simulink model "walkingRobotRL3D"  (R2020b)
settings: Solver=ode23t  StartTime=0.0  StopTime=Tf  RelTol=1e-2  EnableMultiTasking=on
PreLoadFcn:
  | robotParametersRL
undefined symbols (not defined in the file): agent, ankleD_pitch_jointMAX, ankleD_pitch_jointMIN, ankleD_roll_jointMAX, ankleD_roll_jointMIN, ankleI_pitch_jointMAX, ankleI_pitch_jointMIN, ankleI_roll_jointMAX, ankleI_roll_jointMIN, getSampleTime, height_plane, hipD_pitch_jointMAX, hipD_pitch_jointMIN, hipD_roll_jointMAX, hipD_roll_jointMIN, hipI_pitch_jointMAX, hipI_pitch_jointMIN, hipI_roll_jointMAX, hipI_roll_jointMIN, init_angs_L, init_angs_R, init_height, joint_damping, joint_limit_damping, joint_limit_stiffness, joint_stiffness, kneeD_jointMAX, kneeD_jointMIN, kneeI_jointMAX, kneeI_jointMIN, lower_leg_I0, lower_leg_length, lower_leg_mass, lower_leg_x, lower_leg_y, muscle_nominal_length, p10_ankleD_roll, plane_x, plane_y, regulator_type, tau, Tf, torso_height, torso_length, torso_offset_x, torso_offset_z, torso_width, torso_x, torso_y, torso_z, Ts, upper_leg_I0, upper_leg_length, upper_leg_mass, upper_leg_x, upper_leg_y, v10_ankleD_pitch, v10_ankleD_roll, v10_ankleI_pitch, v10_ankleI_roll ... (+41)
libraries: sm_lib x222, simulink x183, nesl_utility x130, walkingRobotUtils x69, rllib x2
(part 13 of 24)

== system walkingRobotRL3D/Walking Robot2/Robot Leg R1/Knee Joint ==
  t : Inport
  Bus Creator : BusCreator  Inputs=3
  PS-Simulink Converter1 : nesl_utility/PS-Simulink Converter  PhysicalDomain=network_engine_domain  SubClassName=ps_output  LeftPortType=input  RightPortType=output  PseudoPeriodic=off  Frequencies=[]  Unit=N*m  AffineConversion=off
  PS-Simulink Converter2 : nesl_utility/PS-Simulink Converter  PhysicalDomain=network_engine_domain  SubClassName=ps_output  LeftPortType=input  RightPortType=output  PseudoPeriodic=off  Frequencies=[]  Unit=rad/s  AffineConversion=off
  Revolute Joint : sm_lib/Joints/Revolute Joint  JointMode=Normal  SenseConstraintForce=off  SenseConstraintForceX=off  SenseConstraintForceY=off  SenseConstraintForceZ=off  SenseConstraintTorque=off  SenseConstraintTorqueX=off  SenseConstraintTorqueY=off  SenseConstraintTorqueZ=off  SenseTotalForce=off  SenseTotalForceX=off  SenseTotalForceY=off  SenseTotalForceZ=off  SenseTotalTorque=off  SenseTotalTorqueX=off  SenseTotalTorqueY=off  SenseTotalTorqueZ=off  CompositeWrenchDir=FollowerOnBase  CompositeWrenchFrame=BaseFrame  EquilibriumPosition=eqAngle  EquilibriumPositionUnits=rad  SpringStiffness=k  SpringStiffnessUnits=N*m/rad  DampingCoefficient=d  DampingCoefficientUnits=N*m/(rad/s)  TorqueActuationMode=ComputedTorque  MotionActuationMode=InputMotion  SensePosition=off  SenseVelocity=on  SenseAcceleration=off  SenseTorqueForce=on  SenseLowerLimitTorqueForce=off  SenseUpperLimitTorqueForce=off  LowerLimitSpecify=on  LowerLimitBound=lowerLimit  LowerLimitBoundUnits=rad  LowerLimitStiffness=jointLimitStiffness  LowerLimitStiffnessUnits=N*m/rad  LowerLimitDamping=jointLimitDamping  LowerLimitDampingUnits=N*m/(rad/s)  LowerLimitTransitionRegionWidth=1  LowerLimitTransitionRegionWidthUnits=deg  UpperLimitSpecify=on  UpperLimitBound=upperLimit  UpperLimitBoundUnits=rad  UpperLimitStiffness=jointLimitStiffness  UpperLimitStiffnessUnits=N*m/rad  UpperLimitDamping=jointLimitDamping  UpperLimitDampingUnits=N*m/(rad/s)  UpperLimitTransitionRegionWidth=1  UpperLimitTransitionRegionWidthUnits=deg  PositionTargetSpecify=on  PositionTargetPriority=High  PositionTargetValue=initAngle  PositionTargetValueUnits=rad  VelocityTargetSpecify=off  VelocityTargetPriority=High  VelocityTargetValue=0  VelocityTargetValueUnits=deg/s
  Simulink-PS Converter : nesl_utility/Simulink-PS Converter  PhysicalDomain=network_engine_domain  SubClassName=ps_input  LeftPortType=input  RightPortType=output  PseudoPeriodic=off  Frequencies=[]  NoiseDistribution=none  NoiseParameters=[]  Unit=rad  AffineConversion=off  FilteringAndDerivatives=filter  SimscapeFilterOrder=2  InputFilterTimeConstant=motion_time_constant  UdotUserProvided=0
  B : PMIOPort  Side=Left
  F : PMIOPort  Port=2  Side=Right
  meas : Outport  VectorParamsAs1DForOutWhenUnconnected=off
  wires:
  PS-Simulink Converter1/1 -> Bus Creator/2  "torque"
  Bus Creator/1 -> meas/1
  t/1 -> Bus Creator/1, Simulink-PS Converter/1  "angle"
  PS-Simulink Converter2/1 -> Bus Creator/3  "speed"
  connections:
  Revolute Joint/LConn1 -- B/RConn1
  Revolute Joint/RConn1 -- F/RConn1
  Simulink-PS Converter/RConn1 -- Revolute Joint/LConn2
  Revolute Joint/RConn2 -- PS-Simulink Converter2/LConn1
  Revolute Joint/RConn3 -- PS-Simulink Converter1/LConn1

== system walkingRobotRL3D/Walking Robot2/Sensors/Calculate Actuator Power 3D ==
  meas : Inport
  Add : Sum  Inputs=5
  Bus Selector : BusSelector  OutputSignals=ankle_roll_angle,ankle_roll_speed,ankle_pitch_angle,ankle_pitch_speed,knee_angle,knee_speed,hip_roll_angle,hip_roll_speed,hip_pitch_angle,hip_pitch_speed
  Product{,1..4} (5 alike) : Product
  P : Outport  VectorParamsAs1DForOutWhenUnconnected=off
  wires:
  meas/1 -> Bus Selector/1
  Product2/1 -> Add/4
  Product1/1 -> Add/2
  Product/1 -> Add/1
  Add/1 -> P/1
  Bus Selector/1 -> Product/1  "<ankle_roll_angle>"
  Bus Selector/2 -> Product/2  "<ankle_roll_speed>"
  Bus Selector/3 -> Product1/1  "<ankle_pitch_angle>"
  Bus Selector/4 -> Product1/2  "<ankle_pitch_speed>"
  Bus Selector/5 -> Product3/1  "<knee_angle>"
  Bus Selector/6 -> Product3/2  "<knee_speed>"
  Bus Selector/7 -> Product2/1  "<hip_roll_angle>"
  Bus Selector/8 -> Product2/2  "<hip_roll_speed>"
  Bus Selector/10 -> Product4/2  "<hip_pitch_speed>"
  Bus Selector/9 -> Product4/1  "<hip_pitch_angle>"
  Product4/1 -> Add/5
  Product3/1 -> Add/3

== system walkingRobotRL3D/Walking Robot2/Sensors/Calculate Actuator Power 3D1 ==
  meas : Inport
  Add : Sum  Inputs=5
  Bus Selector : BusSelector  OutputSignals=ankle_roll_angle,ankle_roll_speed,ankle_pitch_angle,ankle_pitch_speed,knee_angle,knee_speed,hip_roll_angle,hip_roll_speed,hip_pitch_angle,hip_pitch_speed
  Product{,1..4} (5 alike) : Product
  P : Outport  VectorParamsAs1DForOutWhenUnconnected=off
  wires:
  Product3/1 -> Add/3
  Product4/1 -> Add/5
  Bus Selector/9 -> Product4/1  "<hip_pitch_angle>"
  Bus Selector/10 -> Product4/2  "<hip_pitch_speed>"
  Bus Selector/8 -> Product2/2  "<hip_roll_speed>"
  Bus Selector/7 -> Product2/1  "<hip_roll_angle>"
  Bus Selector/6 -> Product3/2  "<knee_speed>"
  Bus Selector/5 -> Product3/1  "<knee_angle>"
  Bus Selector/4 -> Product1/2  "<ankle_pitch_speed>"
  Bus Selector/3 -> Product1/1  "<ankle_pitch_angle>"
  Bus Selector/2 -> Product/2  "<ankle_roll_speed>"
  Bus Selector/1 -> Product/1  "<ankle_roll_angle>"
  Add/1 -> P/1
  Product/1 -> Add/1
  Product1/1 -> Add/2
  Product2/1 -> Add/4
  meas/1 -> Bus Selector/1

== system walkingRobotRL3D/Walking Robot33/DYNAMIC MODEL OF PAM FOR LEFT LEG/Dynamic Model Antagonisitic PAM1 ==
  V1 : Inport
  V2 : Inport  Port=2
  Abs : Abs  Commented=through
  Constant : Constant
  Constant1 : Constant
  F(x,P) mode (Muscles 1) : MATLAB Function  TreatAsAtomicUnit=on
  F(x,P) mode (Muscles 1)1 : MATLAB Function  TreatAsAtomicUnit=on
  Proportional Regulator (Muscles 1) : MATLAB Function  TreatAsAtomicUnit=on
  Proportional Regulator (Muscles 2) : MATLAB Function  TreatAsAtomicUnit=on
  Spring and damping model : Subsystem
  F1 : Outport
  F2 : Outport  Port=2
  wires:
  Constant1/1 -> Proportional Regulator (Muscles 2)/2(reg_type)
  F(x,P) mode (Muscles 1)/1(F1) -> Spring and damping model/1(F1), F1/1
  Proportional Regulator (Muscles 2)/1(p1) -> Spring and damping model/4(P2), F(x,P) mode (Muscles 1)1/1(P2)
  Proportional Regulator (Muscles 1)/1(p1) -> Spring and damping model/3(P1), F(x,P) mode (Muscles 1)/1(P1)
  Spring and damping model/1(x2) -> F(x,P) mode (Muscles 1)1/2(x_muscle2)
  F(x,P) mode (Muscles 1)1/1(F2) -> Abs/1
  Constant/1 -> Proportional Regulator (Muscles 1)/2(reg_type)
  V2/1 -> Proportional Regulator (Muscles 2)/1(V1)
  V1/1 -> Proportional Regulator (Muscles 1)/1(V1)
  Abs/1 -> F2/1, Spring and damping model/2(F2)
  Spring and damping model/2(x1) -> F(x,P) mode (Muscles 1)/2(x_muscle1)

== system walkingRobotRL3D/Walking Robot33/DYNAMIC MODEL OF PAM FOR LEFT LEG/Dynamic Model Antagonisitic PAM2 ==
  V1 : Inport
  V2 : Inport  Port=2
  Abs : Abs  Commented=through
  Constant : Constant
  Constant1 : Constant
  F(x,P) mode (Muscles 1) : MATLAB Function  TreatAsAtomicUnit=on
  F(x,P) mode (Muscles 1)1 : MATLAB Function  TreatAsAtomicUnit=on
  Proportional Regulator (Muscles 1) : MATLAB Function  TreatAsAtomicUnit=on
  Proportional Regulator (Muscles 2) : MATLAB Function  TreatAsAtomicUnit=on
  Spring and damping model : Subsystem
  F1 : Outport
  F2 : Outport  Port=2
  wires:
  Constant1/1 -> Proportional Regulator (Muscles 2)/2(reg_type)
  F(x,P) mode (Muscles 1)/1(F1) -> Spring and damping model/1(F1), F1/1
  Proportional Regulator (Muscles 2)/1(p1) -> Spring and damping model/4(P2), F(x,P) mode (Muscles 1)1/1(P2)
  Proportional Regulator (Muscles 1)/1(p1) -> Spring and damping model/3(P1), F(x,P) mode (Muscles 1)/1(P1)
  Spring and damping model/1(x2) -> F(x,P) mode (Muscles 1)1/2(x_muscle2)
  F(x,P) mode (Muscles 1)1/1(F2) -> Abs/1
  Constant/1 -> Proportional Regulator (Muscles 1)/2(reg_type)
  V2/1 -> Proportional Regulator (Muscles 2)/1(V1)
  V1/1 -> Proportional Regulator (Muscles 1)/1(V1)
  Abs/1 -> F2/1, Spring and damping model/2(F2)
  Spring and damping model/2(x1) -> F(x,P) mode (Muscles 1)/2(x_muscle1)

== system walkingRobotRL3D/Walking Robot33/DYNAMIC MODEL OF PAM FOR LEFT LEG/Dynamic Model Antagonisitic PAM3 ==
  V1 : Inport
  V2 : Inport  Port=2
  Abs : Abs  Commented=through
  Constant : Constant
  Constant1 : Constant
  F(x,P) mode (Muscles 1) : MATLAB Function  TreatAsAtomicUnit=on
  F(x,P) mode (Muscles 1)1 : MATLAB Function  TreatAsAtomicUnit=on
  Proportional Regulator (Muscles 1) : MATLAB Function  TreatAsAtomicUnit=on
  Proportional Regulator (Muscles 2) : MATLAB Function  TreatAsAtomicUnit=on
  Spring and damping model : Subsystem
  F1 : Outport
  F2 : Outport  Port=2
  wires:
  Constant1/1 -> Proportional Regulator (Muscles 2)/2(reg_type)
  F(x,P) mode (Muscles 1)/1(F1) -> Spring and damping model/1(F1), F1/1
  Proportional Regulator (Muscles 2)/1(p1) -> Spring and damping model/4(P2), F(x,P) mode (Muscles 1)1/1(P2)
  Proportional Regulator (Muscles 1)/1(p1) -> Spring and damping model/3(P1), F(x,P) mode (Muscles 1)/1(P1)
  Spring and damping model/1(x2) -> F(x,P) mode (Muscles 1)1/2(x_muscle2)
  F(x,P) mode (Muscles 1)1/1(F2) -> Abs/1
  Constant/1 -> Proportional Regulator (Muscles 1)/2(reg_type)
  V2/1 -> Proportional Regulator (Muscles 2)/1(V1)
  V1/1 -> Proportional Regulator (Muscles 1)/1(V1)
  Abs/1 -> F2/1, Spring and damping model/2(F2)
  Spring and damping model/2(x1) -> F(x,P) mode (Muscles 1)/2(x_muscle1)

== system walkingRobotRL3D/Walking Robot33/DYNAMIC MODEL OF PAM FOR LEFT LEG/Dynamic Model Antagonisitic PAM4 ==
  V1 : Inport
  V2 : Inport  Port=2
  Abs : Abs  Commented=through
  Constant : Constant
  Constant1 : Constant
  F(x,P) mode (Muscles 1) : MATLAB Function  TreatAsAtomicUnit=on
  F(x,P) mode (Muscles 1)1 : MATLAB Function  TreatAsAtomicUnit=on
  Proportional Regulator (Muscles 1) : MATLAB Function  TreatAsAtomicUnit=on
  Proportional Regulator (Muscles 2) : MATLAB Function  TreatAsAtomicUnit=on
  Spring and damping model : Subsystem
  F1 : Outport
  F2 : Outport  Port=2
  wires:
  Constant1/1 -> Proportional Regulator (Muscles 2)/2(reg_type)
  F(x,P) mode (Muscles 1)/1(F1) -> Spring and damping model/1(F1), F1/1
  Proportional Regulator (Muscles 2)/1(p1) -> Spring and damping model/4(P2), F(x,P) mode (Muscles 1)1/1(P2)
  Proportional Regulator (Muscles 1)/1(p1) -> Spring and damping model/3(P1), F(x,P) mode (Muscles 1)/1(P1)
  Spring and damping model/1(x2) -> F(x,P) mode (Muscles 1)1/2(x_muscle2)
  F(x,P) mode (Muscles 1)1/1(F2) -> Abs/1
  Constant/1 -> Proportional Regulator (Muscles 1)/2(reg_type)
  V2/1 -> Proportional Regulator (Muscles 2)/1(V1)
  V1/1 -> Proportional Regulator (Muscles 1)/1(V1)
  Abs/1 -> F2/1, Spring and damping model/2(F2)
  Spring and damping model/2(x1) -> F(x,P) mode (Muscles 1)/2(x_muscle1)

== system walkingRobotRL3D/Walking Robot33/DYNAMIC MODEL OF PAM FOR LEFT LEG/Dynamic Model Antagonisitic PAM5 ==
  V1 : Inport
  V2 : Inport  Port=2
  Abs : Abs  Commented=through
  Constant : Constant
  Constant1 : Constant
  F(x,P) mode (Muscles 1) : MATLAB Function  TreatAsAtomicUnit=on
  F(x,P) mode (Muscles 1)1 : MATLAB Function  TreatAsAtomicUnit=on
  Proportional Regulator (Muscles 1) : MATLAB Function  TreatAsAtomicUnit=on
  Proportional Regulator (Muscles 2) : MATLAB Function  TreatAsAtomicUnit=on
  Spring and damping model : Subsystem
  F1 : Outport
  F2 : Outport  Port=2
  wires:
  Constant1/1 -> Proportional Regulator (Muscles 2)/2(reg_type)
  F(x,P) mode (Muscles 1)/1(F1) -> Spring and damping model/1(F1), F1/1
  Proportional Regulator (Muscles 2)/1(p1) -> Spring and damping model/4(P2), F(x,P) mode (Muscles 1)1/1(P2)
  Proportional Regulator (Muscles 1)/1(p1) -> Spring and damping model/3(P1), F(x,P) mode (Muscles 1)/1(P1)
  Spring and damping model/1(x2) -> F(x,P) mode (Muscles 1)1/2(x_muscle2)
  F(x,P) mode (Muscles 1)1/1(F2) -> Abs/1
  Constant/1 -> Proportional Regulator (Muscles 1)/2(reg_type)
  V2/1 -> Proportional Regulator (Muscles 2)/1(V1)
  V1/1 -> Proportional Regulator (Muscles 1)/1(V1)
  Abs/1 -> F2/1, Spring and damping model/2(F2)
  Spring and damping model/2(x1) -> F(x,P) mode (Muscles 1)/2(x_muscle1)

== system walkingRobotRL3D/Walking Robot33/DYNAMIC MODEL OF PAM FOR RIGHT LEG/Dynamic Model Antagonisitic PAM1 ==
  V1 : Inport
  V2 : Inport  Port=2
  Abs : Abs  Commented=through
  Constant : Constant
  Constant1 : Constant
  F(x,P) mode (Muscles 1) : MATLAB Function  TreatAsAtomicUnit=on
  F(x,P) mode (Muscles 1)1 : MATLAB Function  TreatAsAtomicUnit=on
  Proportional Regulator (Muscles 1) : MATLAB Function  TreatAsAtomicUnit=on
  Proportional Regulator (Muscles 2) : MATLAB Function  TreatAsAtomicUnit=on
  Spring and damping model : Subsystem
  F1 : Outport
  F2 : Outport  Port=2
  wires:
  Constant1/1 -> Proportional Regulator (Muscles 2)/2(reg_type)
  F(x,P) mode (Muscles 1)/1(F1) -> Spring and damping model/1(F1), F1/1
  Proportional Regulator (Muscles 2)/1(p1) -> Spring and damping model/4(P2), F(x,P) mode (Muscles 1)1/1(P2)
  Proportional Regulator (Muscles 1)/1(p1) -> Spring and damping model/3(P1), F(x,P) mode (Muscles 1)/1(P1)
  Spring and damping model/1(x2) -> F(x,P) mode (Muscles 1)1/2(x_muscle2)
  F(x,P) mode (Muscles 1)1/1(F2) -> Abs/1
  Constant/1 -> Proportional Regulator (Muscles 1)/2(reg_type)
  V2/1 -> Proportional Regulator (Muscles 2)/1(V1)
  V1/1 -> Proportional Regulator (Muscles 1)/1(V1)
  Abs/1 -> F2/1, Spring and damping model/2(F2)
  Spring and damping model/2(x1) -> F(x,P) mode (Muscles 1)/2(x_muscle1)

== system walkingRobotRL3D/Walking Robot33/DYNAMIC MODEL OF PAM FOR RIGHT LEG/Dynamic Model Antagonisitic PAM2 ==
  V1 : Inport
  V2 : Inport  Port=2
  Abs : Abs  Commented=through
  Constant : Constant
  Constant1 : Constant
  F(x,P) mode (Muscles 1) : MATLAB Function  TreatAsAtomicUnit=on
  F(x,P) mode (Muscles 1)1 : MATLAB Function  TreatAsAtomicUnit=on
  Proportional Regulator (Muscles 1) : MATLAB Function  TreatAsAtomicUnit=on
  Proportional Regulator (Muscles 2) : MATLAB Function  TreatAsAtomicUnit=on
  Spring and damping model : Subsystem
  F1 : Outport
  F2 : Outport  Port=2
  wires:
  Constant1/1 -> Proportional Regulator (Muscles 2)/2(reg_type)
  F(x,P) mode (Muscles 1)/1(F1) -> Spring and damping model/1(F1), F1/1
  Proportional Regulator (Muscles 2)/1(p1) -> Spring and damping model/4(P2), F(x,P) mode (Muscles 1)1/1(P2)
  Proportional Regulator (Muscles 1)/1(p1) -> Spring and damping model/3(P1), F(x,P) mode (Muscles 1)/1(P1)
  Spring and damping model/1(x2) -> F(x,P) mode (Muscles 1)1/2(x_muscle2)
  F(x,P) mode (Muscles 1)1/1(F2) -> Abs/1
  Constant/1 -> Proportional Regulator (Muscles 1)/2(reg_type)
  V2/1 -> Proportional Regulator (Muscles 2)/1(V1)
  V1/1 -> Proportional Regulator (Muscles 1)/1(V1)
  Abs/1 -> F2/1, Spring and damping model/2(F2)
  Spring and damping model/2(x1) -> F(x,P) mode (Muscles 1)/2(x_muscle1)

== system walkingRobotRL3D/Walking Robot33/DYNAMIC MODEL OF PAM FOR RIGHT LEG/Dynamic Model Antagonisitic PAM3 ==
  V1 : Inport
  V2 : Inport  Port=2
  Abs : Abs  Commented=through
  Constant : Constant
  Constant1 : Constant
  F(x,P) mode (Muscles 1) : MATLAB Function  TreatAsAtomicUnit=on
  F(x,P) mode (Muscles 1)1 : MATLAB Function  TreatAsAtomicUnit=on
  Proportional Regulator (Muscles 1) : MATLAB Function  TreatAsAtomicUnit=on
  Proportional Regulator (Muscles 2) : MATLAB Function  TreatAsAtomicUnit=on
  Spring and damping model : Subsystem
  F1 : Outport
  F2 : Outport  Port=2
  wires:
  Constant1/1 -> Proportional Regulator (Muscles 2)/2(reg_type)
  F(x,P) mode (Muscles 1)/1(F1) -> Spring and damping model/1(F1), F1/1
  Proportional Regulator (Muscles 2)/1(p1) -> Spring and damping model/4(P2), F(x,P) mode (Muscles 1)1/1(P2)
  Proportional Regulator (Muscles 1)/1(p1) -> Spring and damping model/3(P1), F(x,P) mode (Muscles 1)/1(P1)
  Spring and damping model/1(x2) -> F(x,P) mode (Muscles 1)1/2(x_muscle2)
  F(x,P) mode (Muscles 1)1/1(F2) -> Abs/1
  Constant/1 -> Proportional Regulator (Muscles 1)/2(reg_type)
  V2/1 -> Proportional Regulator (Muscles 2)/1(V1)
  V1/1 -> Proportional Regulator (Muscles 1)/1(V1)
  Abs/1 -> F2/1, Spring and damping model/2(F2)
  Spring and damping model/2(x1) -> F(x,P) mode (Muscles 1)/2(x_muscle1)

== system walkingRobotRL3D/Walking Robot33/DYNAMIC MODEL OF PAM FOR RIGHT LEG/Dynamic Model Antagonisitic PAM4 ==
  V1 : Inport
  V2 : Inport  Port=2
  Abs : Abs  Commented=through
  Constant : Constant
  Constant1 : Constant
  F(x,P) mode (Muscles 1) : MATLAB Function  TreatAsAtomicUnit=on
  F(x,P) mode (Muscles 1)1 : MATLAB Function  TreatAsAtomicUnit=on
  Proportional Regulator (Muscles 1) : MATLAB Function  TreatAsAtomicUnit=on
  Proportional Regulator (Muscles 2) : MATLAB Function  TreatAsAtomicUnit=on
  Spring and damping model : Subsystem
  F1 : Outport
  F2 : Outport  Port=2
  wires:
  Constant1/1 -> Proportional Regulator (Muscles 2)/2(reg_type)
  F(x,P) mode (Muscles 1)/1(F1) -> Spring and damping model/1(F1), F1/1
  Proportional Regulator (Muscles 2)/1(p1) -> Spring and damping model/4(P2), F(x,P) mode (Muscles 1)1/1(P2)
  Proportional Regulator (Muscles 1)/1(p1) -> Spring and damping model/3(P1), F(x,P) mode (Muscles 1)/1(P1)
  Spring and damping model/1(x2) -> F(x,P) mode (Muscles 1)1/2(x_muscle2)
  F(x,P) mode (Muscles 1)1/1(F2) -> Abs/1
  Constant/1 -> Proportional Regulator (Muscles 1)/2(reg_type)
  V2/1 -> Proportional Regulator (Muscles 2)/1(V1)
  V1/1 -> Proportional Regulator (Muscles 1)/1(V1)
  Abs/1 -> F2/1, Spring and damping model/2(F2)
  Spring and damping model/2(x1) -> F(x,P) mode (Muscles 1)/2(x_muscle1)

== system walkingRobotRL3D/Walking Robot33/DYNAMIC MODEL OF PAM FOR RIGHT LEG/Dynamic Model Antagonisitic PAM5 ==
  V1 : Inport
  V2 : Inport  Port=2
  Abs : Abs  Commented=through
  Constant : Constant
  Constant1 : Constant
  F(x,P) mode (Muscles 1) : MATLAB Function  TreatAsAtomicUnit=on
  F(x,P) mode (Muscles 1)1 : MATLAB Function  TreatAsAtomicUnit=on
  Proportional Regulator (Muscles 1) : MATLAB Function  TreatAsAtomicUnit=on
  Proportional Regulator (Muscles 2) : MATLAB Function  TreatAsAtomicUnit=on
  Spring and damping model : Subsystem
  F1 : Outport
  F2 : Outport  Port=2
  wires:
  Constant1/1 -> Proportional Regulator (Muscles 2)/2(reg_type)
  F(x,P) mode (Muscles 1)/1(F1) -> Spring and damping model/1(F1), F1/1
  Proportional Regulator (Muscles 2)/1(p1) -> Spring and damping model/4(P2), F(x,P) mode (Muscles 1)1/1(P2)
  Proportional Regulator (Muscles 1)/1(p1) -> Spring and damping model/3(P1), F(x,P) mode (Muscles 1)/1(P1)
  Spring and damping model/1(x2) -> F(x,P) mode (Muscles 1)1/2(x_muscle2)
  F(x,P) mode (Muscles 1)1/1(F2) -> Abs/1
  Constant/1 -> Proportional Regulator (Muscles 1)/2(reg_type)
  V2/1 -> Proportional Regulator (Muscles 2)/1(V1)
  V1/1 -> Proportional Regulator (Muscles 1)/1(V1)
  Abs/1 -> F2/1, Spring and damping model/2(F2)
  Spring and damping model/2(x1) -> F(x,P) mode (Muscles 1)/2(x_muscle1)

== system walkingRobotRL3D/Walking Robot33/Sensors/Calculate Actuator Power 3D ==
  meas : Inport
  Add : Sum  Inputs=5
  Bus Selector : BusSelector  OutputSignals=ankle_roll_angle,ankle_roll_speed,ankle_pitch_angle,ankle_pitch_speed,knee_angle,knee_speed,hip_roll_angle,hip_roll_speed,hip_pitch_angle,hip_pitch_speed
  Product{,1..4} (5 alike) : Product
  P : Outport  VectorParamsAs1DForOutWhenUnconnected=off
  wires:
  meas/1 -> Bus Selector/1
  Product2/1 -> Add/4
  Product1/1 -> Add/2
  Product/1 -> Add/1
  Add/1 -> P/1
  Bus Selector/1 -> Product/1  "<ankle_roll_angle>"
  Bus Selector/2 -> Product/2  "<ankle_roll_speed>"
  Bus Selector/3 -> Product1/1  "<ankle_pitch_angle>"
  Bus Selector/4 -> Product1/2  "<ankle_pitch_speed>"
  Bus Selector/5 -> Product3/1  "<knee_angle>"
  Bus Selector/6 -> Product3/2  "<knee_speed>"
  Bus Selector/7 -> Product2/1  "<hip_roll_angle>"
  Bus Selector/8 -> Product2/2  "<hip_roll_speed>"
  Bus Selector/10 -> Product4/2  "<hip_pitch_speed>"
  Bus Selector/9 -> Product4/1  "<hip_pitch_angle>"
  Product4/1 -> Add/5
  Product3/1 -> Add/3

== system walkingRobotRL3D/Walking Robot33/Sensors/Calculate Actuator Power 3D1 ==
  meas : Inport
  Add : Sum  Inputs=5
  Bus Selector : BusSelector  OutputSignals=ankle_roll_angle,ankle_roll_speed,ankle_pitch_angle,ankle_pitch_speed,knee_angle,knee_speed,hip_roll_angle,hip_roll_speed,hip_pitch_angle,hip_pitch_speed
  Product{,1..4} (5 alike) : Product
  P : Outport  VectorParamsAs1DForOutWhenUnconnected=off
  wires:
  Product3/1 -> Add/3
  Product4/1 -> Add/5
  Bus Selector/9 -> Product4/1  "<hip_pitch_angle>"
  Bus Selector/10 -> Product4/2  "<hip_pitch_speed>"
  Bus Selector/8 -> Product2/2  "<hip_roll_speed>"
  Bus Selector/7 -> Product2/1  "<hip_roll_angle>"
  Bus Selector/6 -> Product3/2  "<knee_speed>"
  Bus Selector/5 -> Product3/1  "<knee_angle>"
  Bus Selector/4 -> Product1/2  "<ankle_pitch_speed>"
  Bus Selector/3 -> Product1/1  "<ankle_pitch_angle>"
  Bus Selector/2 -> Product/2  "<ankle_roll_speed>"
  Bus Selector/1 -> Product/1  "<ankle_roll_angle>"
  Add/1 -> P/1
  Product/1 -> Add/1
  Product1/1 -> Add/2
  Product2/1 -> Add/4
  meas/1 -> Bus Selector/1

== system walkingRobotRL3D/Walking Robot/DYNAMIC MODEL OF PAM FOR LEFT LEG/Dynamic Model Antagonisitic PAM1/Spring and damping model ==
  F1 : Inport
  F2 : Inport  Port=2
  P1 : Inport  Port=3
  P2 : Inport  Port=4
  Dynamic muscle 2 : Subsystem
  Dynamics muscle 1 : Subsystem
  S(P),D(P) : MATLAB Function  TreatAsAtomicUnit=on
  Unit Delay : UnitDelay  SampleTime=-1  HasFrameUpgradeWarning=on
  Unit Delay1 : UnitDelay  SampleTime=-1  HasFrameUpgradeWarning=on
  Unit Delay2 : UnitDelay  Commented=through  SampleTime=-1  HasFrameUpgradeWarning=on
  Unit Delay3 : UnitDelay  Commented=through  SampleTime=-1  HasFrameUpgradeWarning=on
  x1(m)->x1(%) : Gain  Gain=100/muscle_nominal_length
  x2(m)->x2(%) : Gain  Gain=100/muscle_nominal_length
  x2 : Outport
  x1 : Outport  Port=2
  wires:
  Dynamics muscle 1/1(R1) -> Unit Delay/1
  F1/1 -> Unit Delay2/1
  Dynamic muscle 2/2(x2) -> x2(m)->x2(%)/1
  Dynamics muscle 1/2(x1) -> x1(m)->x1(%)/1
  P1/1 -> S(P),D(P)/1(P1)
  x2(m)->x2(%)/1 -> x2/1
  x1(m)->x1(%)/1 -> x1/1
  F2/1 -> Unit Delay3/1
  P2/1 -> S(P),D(P)/2(P2)
  Unit Delay/1 -> Dynamic muscle 2/2(R1)
  Dynamic muscle 2/1(R2) -> Unit Delay1/1
  Unit Delay1/1 -> Dynamics muscle 1/3(R2)
  Unit Delay2/1 -> Dynamics muscle 1/1(F1)
  Unit Delay3/1 -> Dynamic muscle 2/3(F2)
  S(P),D(P)/2(D1) -> Dynamics muscle 1/4(D1)
  S(P),D(P)/3(S2) -> Dynamic muscle 2/1(S2)
  S(P),D(P)/4(D2) -> Dynamic muscle 2/4(D2)
  S(P),D(P)/1(S1) -> Dynamics muscle 1/2(S1)

== system walkingRobotRL3D/Walking Robot/DYNAMIC MODEL OF PAM FOR LEFT LEG/Dynamic Model Antagonisitic PAM2/Spring and damping model ==
  F1 : Inport
  F2 : Inport  Port=2
  P1 : Inport  Port=3
  P2 : Inport  Port=4
  Dynamic muscle 2 : Subsystem
  Dynamics muscle 1 : Subsystem
  S(P),D(P) : MATLAB Function  TreatAsAtomicUnit=on
  Unit Delay : UnitDelay  SampleTime=-1  HasFrameUpgradeWarning=on
  Unit Delay1 : UnitDelay  SampleTime=-1  HasFrameUpgradeWarning=on
  Unit Delay2 : UnitDelay  Commented=through  SampleTime=-1  HasFrameUpgradeWarning=on
  Unit Delay3 : UnitDelay  Commented=through  SampleTime=-1  HasFrameUpgradeWarning=on
  x1(m)->x1(%) : Gain  Gain=100/muscle_nominal_length
  x2(m)->x2(%) : Gain  Gain=100/muscle_nominal_length
  x2 : Outport
  x1 : Outport  Port=2
  wires:
  Dynamics muscle 1/1(R1) -> Unit Delay/1
  F1/1 -> Unit Delay2/1
  Dynamic muscle 2/2(x2) -> x2(m)->x2(%)/1
  Dynamics muscle 1/2(x1) -> x1(m)->x1(%)/1
  P1/1 -> S(P),D(P)/1(P1)
  x2(m)->x2(%)/1 -> x2/1
  x1(m)->x1(%)/1 -> x1/1
  F2/1 -> Unit Delay3/1
  P2/1 -> S(P),D(P)/2(P2)
  Unit Delay/1 -> Dynamic muscle 2/2(R1)
  Dynamic muscle 2/1(R2) -> Unit Delay1/1
  Unit Delay1/1 -> Dynamics muscle 1/3(R2)
  Unit Delay2/1 -> Dynamics muscle 1/1(F1)
  Unit Delay3/1 -> Dynamic muscle 2/3(F2)
  S(P),D(P)/2(D1) -> Dynamics muscle 1/4(D1)
  S(P),D(P)/3(S2) -> Dynamic muscle 2/1(S2)
  S(P),D(P)/4(D2) -> Dynamic muscle 2/4(D2)
  S(P),D(P)/1(S1) -> Dynamics muscle 1/2(S1)

== system walkingRobotRL3D/Walking Robot/DYNAMIC MODEL OF PAM FOR LEFT LEG/Dynamic Model Antagonisitic PAM3/Spring and damping model ==
  F1 : Inport
  F2 : Inport  Port=2
  P1 : Inport  Port=3
  P2 : Inport  Port=4
  Dynamic muscle 2 : Subsystem
  Dynamics muscle 1 : Subsystem
  S(P),D(P) : MATLAB Function  TreatAsAtomicUnit=on
  Unit Delay : UnitDelay  SampleTime=-1  HasFrameUpgradeWarning=on
  Unit Delay1 : UnitDelay  SampleTime=-1  HasFrameUpgradeWarning=on
  Unit Delay2 : UnitDelay  Commented=through  SampleTime=-1  HasFrameUpgradeWarning=on
  Unit Delay3 : UnitDelay  Commented=through  SampleTime=-1  HasFrameUpgradeWarning=on
  x1(m)->x1(%) : Gain  Gain=100/muscle_nominal_length
  x2(m)->x2(%) : Gain  Gain=100/muscle_nominal_length
  x2 : Outport
  x1 : Outport  Port=2
  wires:
  Dynamics muscle 1/1(R1) -> Unit Delay/1
  F1/1 -> Unit Delay2/1
  Dynamic muscle 2/2(x2) -> x2(m)->x2(%)/1
  Dynamics muscle 1/2(x1) -> x1(m)->x1(%)/1
  P1/1 -> S(P),D(P)/1(P1)
  x2(m)->x2(%)/1 -> x2/1
  x1(m)->x1(%)/1 -> x1/1
  F2/1 -> Unit Delay3/1
  P2/1 -> S(P),D(P)/2(P2)
  Unit Delay/1 -> Dynamic muscle 2/2(R1)
  Dynamic muscle 2/1(R2) -> Unit Delay1/1
  Unit Delay1/1 -> Dynamics muscle 1/3(R2)
  Unit Delay2/1 -> Dynamics muscle 1/1(F1)
  Unit Delay3/1 -> Dynamic muscle 2/3(F2)
  S(P),D(P)/2(D1) -> Dynamics muscle 1/4(D1)
  S(P),D(P)/3(S2) -> Dynamic muscle 2/1(S2)
  S(P),D(P)/4(D2) -> Dynamic muscle 2/4(D2)
  S(P),D(P)/1(S1) -> Dynamics muscle 1/2(S1)

== system walkingRobotRL3D/Walking Robot/DYNAMIC MODEL OF PAM FOR LEFT LEG/Dynamic Model Antagonisitic PAM4/Spring and damping model ==
  F1 : Inport
  F2 : Inport  Port=2
  P1 : Inport  Port=3
  P2 : Inport  Port=4
  Dynamic muscle 2 : Subsystem
  Dynamics muscle 1 : Subsystem
  S(P),D(P) : MATLAB Function  TreatAsAtomicUnit=on
  Unit Delay : UnitDelay  SampleTime=-1  HasFrameUpgradeWarning=on
  Unit Delay1 : UnitDelay  SampleTime=-1  HasFrameUpgradeWarning=on
  Unit Delay2 : UnitDelay  Commented=through  SampleTime=-1  HasFrameUpgradeWarning=on
  Unit Delay3 : UnitDelay  Commented=through  SampleTime=-1  HasFrameUpgradeWarning=on
  x1(m)->x1(%) : Gain  Gain=100/muscle_nominal_length
  x2(m)->x2(%) : Gain  Gain=100/muscle_nominal_length
  x2 : Outport
  x1 : Outport  Port=2
  wires:
  Dynamics muscle 1/1(R1) -> Unit Delay/1
  F1/1 -> Unit Delay2/1
  Dynamic muscle 2/2(x2) -> x2(m)->x2(%)/1
  Dynamics muscle 1/2(x1) -> x1(m)->x1(%)/1
  P1/1 -> S(P),D(P)/1(P1)
  x2(m)->x2(%)/1 -> x2/1
  x1(m)->x1(%)/1 -> x1/1
  F2/1 -> Unit Delay3/1
  P2/1 -> S(P),D(P)/2(P2)
  Unit Delay/1 -> Dynamic muscle 2/2(R1)
  Dynamic muscle 2/1(R2) -> Unit Delay1/1
  Unit Delay1/1 -> Dynamics muscle 1/3(R2)
  Unit Delay2/1 -> Dynamics muscle 1/1(F1)
  Unit Delay3/1 -> Dynamic muscle 2/3(F2)
  S(P),D(P)/2(D1) -> Dynamics muscle 1/4(D1)
  S(P),D(P)/3(S2) -> Dynamic muscle 2/1(S2)
  S(P),D(P)/4(D2) -> Dynamic muscle 2/4(D2)
  S(P),D(P)/1(S1) -> Dynamics muscle 1/2(S1)

== system walkingRobotRL3D/Walking Robot/DYNAMIC MODEL OF PAM FOR LEFT LEG/Dynamic Model Antagonisitic PAM5/Spring and damping model ==
  F1 : Inport
  F2 : Inport  Port=2
  P1 : Inport  Port=3
  P2 : Inport  Port=4
  Dynamic muscle 2 : Subsystem
  Dynamics muscle 1 : Subsystem
  S(P),D(P) : MATLAB Function  TreatAsAtomicUnit=on
  Unit Delay : UnitDelay  SampleTime=-1  HasFrameUpgradeWarning=on
  Unit Delay1 : UnitDelay  SampleTime=-1  HasFrameUpgradeWarning=on
  Unit Delay2 : UnitDelay  Commented=through  SampleTime=-1  HasFrameUpgradeWarning=on
  Unit Delay3 : UnitDelay  Commented=through  SampleTime=-1  HasFrameUpgradeWarning=on
  x1(m)->x1(%) : Gain  Gain=100/muscle_nominal_length
  x2(m)->x2(%) : Gain  Gain=100/muscle_nominal_length
  x2 : Outport
  x1 : Outport  Port=2
  wires:
  Dynamics muscle 1/1(R1) -> Unit Delay/1
  F1/1 -> Unit Delay2/1
  Dynamic muscle 2/2(x2) -> x2(m)->x2(%)/1
  Dynamics muscle 1/2(x1) -> x1(m)->x1(%)/1
  P1/1 -> S(P),D(P)/1(P1)
  x2(m)->x2(%)/1 -> x2/1
  x1(m)->x1(%)/1 -> x1/1
  F2/1 -> Unit Delay3/1
  P2/1 -> S(P),D(P)/2(P2)
  Unit Delay/1 -> Dynamic muscle 2/2(R1)
  Dynamic muscle 2/1(R2) -> Unit Delay1/1
  Unit Delay1/1 -> Dynamics muscle 1/3(R2)
  Unit Delay2/1 -> Dynamics muscle 1/1(F1)
  Unit Delay3/1 -> Dynamic muscle 2/3(F2)
  S(P),D(P)/2(D1) -> Dynamics muscle 1/4(D1)
  S(P),D(P)/3(S2) -> Dynamic muscle 2/1(S2)
  S(P),D(P)/4(D2) -> Dynamic muscle 2/4(D2)
  S(P),D(P)/1(S1) -> Dynamics muscle 1/2(S1)

== system walkingRobotRL3D/Walking Robot/DYNAMIC MODEL OF PAM FOR RIGHT LEG/Dynamic Model Antagonisitic PAM1/Spring and damping model ==
  F1 : Inport
  F2 : Inport  Port=2
  P1 : Inport  Port=3
  P2 : Inport  Port=4
  Dynamic muscle 2 : Subsystem
  Dynamics muscle 1 : Subsystem
  S(P),D(P) : MATLAB Function  TreatAsAtomicUnit=on
  Unit Delay : UnitDelay  SampleTime=-1  HasFrameUpgradeWarning=on
  Unit Delay1 : UnitDelay  SampleTime=-1  HasFrameUpgradeWarning=on
  Unit Delay2 : UnitDelay  Commented=through  SampleTime=-1  HasFrameUpgradeWarning=on
  Unit Delay3 : UnitDelay  Commented=through  SampleTime=-1  HasFrameUpgradeWarning=on
  x1(m)->x1(%) : Gain  Gain=100/muscle_nominal_length
  x2(m)->x2(%) : Gain  Gain=100/muscle_nominal_length
  x2 : Outport
  x1 : Outport  Port=2
  wires:
  Dynamics muscle 1/1(R1) -> Unit Delay/1
  F1/1 -> Unit Delay2/1
  Dynamic muscle 2/2(x2) -> x2(m)->x2(%)/1
  Dynamics muscle 1/2(x1) -> x1(m)->x1(%)/1
  P1/1 -> S(P),D(P)/1(P1)
  x2(m)->x2(%)/1 -> x2/1
  x1(m)->x1(%)/1 -> x1/1
  F2/1 -> Unit Delay3/1
  P2/1 -> S(P),D(P)/2(P2)
  Unit Delay/1 -> Dynamic muscle 2/2(R1)
  Dynamic muscle 2/1(R2) -> Unit Delay1/1
  Unit Delay1/1 -> Dynamics muscle 1/3(R2)
  Unit Delay2/1 -> Dynamics muscle 1/1(F1)
  Unit Delay3/1 -> Dynamic muscle 2/3(F2)
  S(P),D(P)/2(D1) -> Dynamics muscle 1/4(D1)
  S(P),D(P)/3(S2) -> Dynamic muscle 2/1(S2)
  S(P),D(P)/4(D2) -> Dynamic muscle 2/4(D2)
  S(P),D(P)/1(S1) -> Dynamics muscle 1/2(S1)

== system walkingRobotRL3D/Walking Robot/DYNAMIC MODEL OF PAM FOR RIGHT LEG/Dynamic Model Antagonisitic PAM2/Spring and damping model ==
  F1 : Inport
  F2 : Inport  Port=2
  P1 : Inport  Port=3
  P2 : Inport  Port=4
  Dynamic muscle 2 : Subsystem
  Dynamics muscle 1 : Subsystem
  S(P),D(P) : MATLAB Function  TreatAsAtomicUnit=on
  Unit Delay : UnitDelay  SampleTime=-1  HasFrameUpgradeWarning=on
  Unit Delay1 : UnitDelay  SampleTime=-1  HasFrameUpgradeWarning=on
  Unit Delay2 : UnitDelay  Commented=through  SampleTime=-1  HasFrameUpgradeWarning=on
  Unit Delay3 : UnitDelay  Commented=through  SampleTime=-1  HasFrameUpgradeWarning=on
  x1(m)->x1(%) : Gain  Gain=100/muscle_nominal_length
  x2(m)->x2(%) : Gain  Gain=100/muscle_nominal_length
  x2 : Outport
  x1 : Outport  Port=2
  wires:
  Dynamics muscle 1/1(R1) -> Unit Delay/1
  F1/1 -> Unit Delay2/1
  Dynamic muscle 2/2(x2) -> x2(m)->x2(%)/1
  Dynamics muscle 1/2(x1) -> x1(m)->x1(%)/1
  P1/1 -> S(P),D(P)/1(P1)
  x2(m)->x2(%)/1 -> x2/1
  x1(m)->x1(%)/1 -> x1/1
  F2/1 -> Unit Delay3/1
  P2/1 -> S(P),D(P)/2(P2)
  Unit Delay/1 -> Dynamic muscle 2/2(R1)
  Dynamic muscle 2/1(R2) -> Unit Delay1/1
  Unit Delay1/1 -> Dynamics muscle 1/3(R2)
  Unit Delay2/1 -> Dynamics muscle 1/1(F1)
  Unit Delay3/1 -> Dynamic muscle 2/3(F2)
  S(P),D(P)/2(D1) -> Dynamics muscle 1/4(D1)
  S(P),D(P)/3(S2) -> Dynamic muscle 2/1(S2)
  S(P),D(P)/4(D2) -> Dynamic muscle 2/4(D2)
  S(P),D(P)/1(S1) -> Dynamics muscle 1/2(S1)

== system walkingRobotRL3D/Walking Robot/DYNAMIC MODEL OF PAM FOR RIGHT LEG/Dynamic Model Antagonisitic PAM3/Spring and damping model ==
  F1 : Inport
  F2 : Inport  Port=2
  P1 : Inport  Port=3
  P2 : Inport  Port=4
  Dynamic muscle 2 : Subsystem
  Dynamics muscle 1 : Subsystem
  S(P),D(P) : MATLAB Function  TreatAsAtomicUnit=on
  Unit Delay : UnitDelay  SampleTime=-1  HasFrameUpgradeWarning=on
  Unit Delay1 : UnitDelay  SampleTime=-1  HasFrameUpgradeWarning=on
  Unit Delay2 : UnitDelay  Commented=through  SampleTime=-1  HasFrameUpgradeWarning=on
  Unit Delay3 : UnitDelay  Commented=through  SampleTime=-1  HasFrameUpgradeWarning=on
  x1(m)->x1(%) : Gain  Gain=100/muscle_nominal_length
  x2(m)->x2(%) : Gain  Gain=100/muscle_nominal_length
  x2 : Outport
  x1 : Outport  Port=2
  wires:
  Dynamics muscle 1/1(R1) -> Unit Delay/1
  F1/1 -> Unit Delay2/1
  Dynamic muscle 2/2(x2) -> x2(m)->x2(%)/1
  Dynamics muscle 1/2(x1) -> x1(m)->x1(%)/1
  P1/1 -> S(P),D(P)/1(P1)
  x2(m)->x2(%)/1 -> x2/1
  x1(m)->x1(%)/1 -> x1/1
  F2/1 -> Unit Delay3/1
  P2/1 -> S(P),D(P)/2(P2)
  Unit Delay/1 -> Dynamic muscle 2/2(R1)
  Dynamic muscle 2/1(R2) -> Unit Delay1/1
  Unit Delay1/1 -> Dynamics muscle 1/3(R2)
  Unit Delay2/1 -> Dynamics muscle 1/1(F1)
  Unit Delay3/1 -> Dynamic muscle 2/3(F2)
  S(P),D(P)/2(D1) -> Dynamics muscle 1/4(D1)
  S(P),D(P)/3(S2) -> Dynamic muscle 2/1(S2)
  S(P),D(P)/4(D2) -> Dynamic muscle 2/4(D2)
  S(P),D(P)/1(S1) -> Dynamics muscle 1/2(S1)

== system walkingRobotRL3D/Walking Robot/DYNAMIC MODEL OF PAM FOR RIGHT LEG/Dynamic Model Antagonisitic PAM4/Spring and damping model ==
  F1 : Inport
  F2 : Inport  Port=2
  P1 : Inport  Port=3
  P2 : Inport  Port=4
  Dynamic muscle 2 : Subsystem
  Dynamics muscle 1 : Subsystem
  S(P),D(P) : MATLAB Function  TreatAsAtomicUnit=on
  Unit Delay : UnitDelay  SampleTime=-1  HasFrameUpgradeWarning=on
  Unit Delay1 : UnitDelay  SampleTime=-1  HasFrameUpgradeWarning=on
  Unit Delay2 : UnitDelay  Commented=through  SampleTime=-1  HasFrameUpgradeWarning=on
  Unit Delay3 : UnitDelay  Commented=through  SampleTime=-1  HasFrameUpgradeWarning=on
  x1(m)->x1(%) : Gain  Gain=100/muscle_nominal_length
  x2(m)->x2(%) : Gain  Gain=100/muscle_nominal_length
  x2 : Outport
  x1 : Outport  Port=2
  wires:
  Dynamics muscle 1/1(R1) -> Unit Delay/1
  F1/1 -> Unit Delay2/1
  Dynamic muscle 2/2(x2) -> x2(m)->x2(%)/1
  Dynamics muscle 1/2(x1) -> x1(m)->x1(%)/1
  P1/1 -> S(P),D(P)/1(P1)
  x2(m)->x2(%)/1 -> x2/1
  x1(m)->x1(%)/1 -> x1/1
  F2/1 -> Unit Delay3/1
  P2/1 -> S(P),D(P)/2(P2)
  Unit Delay/1 -> Dynamic muscle 2/2(R1)
  Dynamic muscle 2/1(R2) -> Unit Delay1/1
  Unit Delay1/1 -> Dynamics muscle 1/3(R2)
  Unit Delay2/1 -> Dynamics muscle 1/1(F1)
  Unit Delay3/1 -> Dynamic muscle 2/3(F2)
  S(P),D(P)/2(D1) -> Dynamics muscle 1/4(D1)
  S(P),D(P)/3(S2) -> Dynamic muscle 2/1(S2)
  S(P),D(P)/4(D2) -> Dynamic muscle 2/4(D2)
  S(P),D(P)/1(S1) -> Dynamics muscle 1/2(S1)

== system walkingRobotRL3D/Walking Robot/DYNAMIC MODEL OF PAM FOR RIGHT LEG/Dynamic Model Antagonisitic PAM5/Spring and damping model ==
  F1 : Inport
  F2 : Inport  Port=2
  P1 : Inport  Port=3
  P2 : Inport  Port=4
  Dynamic muscle 2 : Subsystem
  Dynamics muscle 1 : Subsystem
  S(P),D(P) : MATLAB Function  TreatAsAtomicUnit=on
  Unit Delay : UnitDelay  SampleTime=-1  HasFrameUpgradeWarning=on
  Unit Delay1 : UnitDelay  SampleTime=-1  HasFrameUpgradeWarning=on
  Unit Delay2 : UnitDelay  Commented=through  SampleTime=-1  HasFrameUpgradeWarning=on
  Unit Delay3 : UnitDelay  Commented=through  SampleTime=-1  HasFrameUpgradeWarning=on
  x1(m)->x1(%) : Gain  Gain=100/muscle_nominal_length
  x2(m)->x2(%) : Gain  Gain=100/muscle_nominal_length
  x2 : Outport
  x1 : Outport  Port=2
  wires:
  Dynamics muscle 1/1(R1) -> Unit Delay/1
  F1/1 -> Unit Delay2/1
  Dynamic muscle 2/2(x2) -> x2(m)->x2(%)/1
  Dynamics muscle 1/2(x1) -> x1(m)->x1(%)/1
  P1/1 -> S(P),D(P)/1(P1)
  x2(m)->x2(%)/1 -> x2/1
  x1(m)->x1(%)/1 -> x1/1
  F2/1 -> Unit Delay3/1
  P2/1 -> S(P),D(P)/2(P2)
  Unit Delay/1 -> Dynamic muscle 2/2(R1)
  Dynamic muscle 2/1(R2) -> Unit Delay1/1
  Unit Delay1/1 -> Dynamics muscle 1/3(R2)
  Unit Delay2/1 -> Dynamics muscle 1/1(F1)
  Unit Delay3/1 -> Dynamic muscle 2/3(F2)
  S(P),D(P)/2(D1) -> Dynamics muscle 1/4(D1)
  S(P),D(P)/3(S2) -> Dynamic muscle 2/1(S2)
  S(P),D(P)/4(D2) -> Dynamic muscle 2/4(D2)
  S(P),D(P)/1(S1) -> Dynamics muscle 1/2(S1)

== system walkingRobotRL3D/Walking Robot (Angle based)/Antagonistic PAM Left Leg/ankleI_pitch PAM/Spring and damping model ==
  F1 : Inport
  F2 : Inport  Port=2
  P1 : Inport  Port=3
  P2 : Inport  Port=4
  Bar->kPa : Gain  Gain=100
  Bar->kPa1 : Gain  Gain=100
  Dynamic muscle 2 : Subsystem
  Dynamics muscle 1 : Subsystem
  Fplot : Scope  NumInputPorts=2
  Pplot : Scope  NumInputPorts=2
  Rplot : Scope  NumInputPorts=2
  Splot : Scope  NumInputPorts=2
  Stimation of spring coefficients : MATLAB Function  TreatAsAtomicUnit=on
  Stimation of spring coefficients1 : MATLAB Function  TreatAsAtomicUnit=on
  Unit Delay{,1..3} (4 alike) : UnitDelay  SampleTime=-1  HasFrameUpgradeWarning=on
  getDeltaXmax : Subsystem
  getDeltaXmax1 : Subsystem
  x(%)->x(m) : Gain  Gain=muscle_nominal_length/100
  x(%)->x(m)1 : Gain  Gain=muscle_nominal_length/100
  x1(m)->x1(%) : Gain  Gain=100/muscle_nominal_length
  x2(m)->x2(%) : Gain  Gain=100/muscle_nominal_length
  xplot : Scope  NumInputPorts=2
  x1 : Outport
  x2 : Outport  Port=2
  wires:
  Dynamics muscle 1/1(R1) -> Unit Delay/1, Unit Delay2/1
  Dynamic muscle 2/1(R2) -> Unit Delay1/1, Unit Delay3/1
  F1/1 -> Stimation of spring coefficients/4(F1), Fplot/1, Dynamics muscle 1/1(F1)
  Dynamic muscle 2/2(x2) -> x2(m)->x2(%)/1
  Dynamics muscle 1/2(x1) -> x1(m)->x1(%)/1
  P1/1 -> Pplot/1, Bar->kPa/1
  Bar->kPa/1 -> Stimation of spring coefficients/1(P1), getDeltaXmax/1(In1)
  P2/1 -> Pplot/2, Bar->kPa1/1
  Bar->kPa1/1 -> getDeltaXmax1/1(In1), Stimation of spring coefficients1/2(P2)
  Stimation of spring coefficients/1(S1) -> Splot/1, Dynamics muscle 1/2(S1)
  Stimation of spring coefficients1/1(S2) -> Splot/2, Dynamic muscle 2/1(S2)
  getDeltaXmax/1(dmax1) -> Stimation of spring coefficients/5(dmax1_per), x(%)->x(m)/1
  x(%)->x(m)/1 -> Stimation of spring coefficients/3(dmax1)
  getDeltaXmax1/1(dmax2) -> Stimation of spring coefficients1/5(dmax2_per), x(%)->x(m)1/1
  x(%)->x(m)1/1 -> Stimation of spring coefficients1/4(dmax2)
  x2(m)->x2(%)/1 -> xplot/2, x2/1
  x1(m)->x1(%)/1 -> xplot/1, x1/1
  F2/1 -> Stimation of spring coefficients1/1(F2), Fplot/2, Dynamic muscle 2/3(F2)
  Unit Delay/1 -> Stimation of spring coefficients1/3(Fload)
  Unit Delay1/1 -> Stimation of spring coefficients/2(Fload)
  Unit Delay2/1 -> Rplot/1, Dynamic muscle 2/2(R1)
  Unit Delay3/1 -> Rplot/2, Dynamics muscle 1/3(R2)

== system walkingRobotRL3D/Walking Robot (Angle based)/Antagonistic PAM Left Leg/ankleI_roll PAM/Spring and damping model ==
  F1 : Inport
  F2 : Inport  Port=2
  P1 : Inport  Port=3
  P2 : Inport  Port=4
  Bar->kPa : Gain  Gain=100
  Bar->kPa1 : Gain  Gain=100
  Dynamic muscle 2 : Subsystem
  Dynamics muscle 1 : Subsystem
  Fplot : Scope  NumInputPorts=2
  Pplot : Scope  NumInputPorts=2
  Rplot : Scope  NumInputPorts=2
  Splot : Scope  NumInputPorts=2
  Stimation of spring coefficients : MATLAB Function  TreatAsAtomicUnit=on
  Stimation of spring coefficients1 : MATLAB Function  TreatAsAtomicUnit=on
  Unit Delay{,1..3} (4 alike) : UnitDelay  SampleTime=-1  HasFrameUpgradeWarning=on
  getDeltaXmax : Subsystem
  getDeltaXmax1 : Subsystem
  x(%)->x(m) : Gain  Gain=muscle_nominal_length/100
  x(%)->x(m)1 : Gain  Gain=muscle_nominal_length/100
  x1(m)->x1(%) : Gain  Gain=100/muscle_nominal_length
  x2(m)->x2(%) : Gain  Gain=100/muscle_nominal_length
  xplot : Scope  NumInputPorts=2
  x1 : Outport
  x2 : Outport  Port=2
  wires:
  Dynamics muscle 1/1(R1) -> Unit Delay/1, Unit Delay2/1
  Dynamic muscle 2/1(R2) -> Unit Delay1/1, Unit Delay3/1
  F1/1 -> Stimation of spring coefficients/4(F1), Fplot/1, Dynamics muscle 1/1(F1)
  Dynamic muscle 2/2(x2) -> x2(m)->x2(%)/1
  Dynamics muscle 1/2(x1) -> x1(m)->x1(%)/1
  P1/1 -> Pplot/1, Bar->kPa/1
  Bar->kPa/1 -> Stimation of spring coefficients/1(P1), getDeltaXmax/1(In1)
  P2/1 -> Pplot/2, Bar->kPa1/1
  Bar->kPa1/1 -> getDeltaXmax1/1(In1), Stimation of spring coefficients1/2(P2)
  Stimation of spring coefficients/1(S1) -> Splot/1, Dynamics muscle 1/2(S1)
  Stimation of spring coefficients1/1(S2) -> Splot/2, Dynamic muscle 2/1(S2)
  getDeltaXmax/1(dmax1) -> Stimation of spring coefficients/5(dmax1_per), x(%)->x(m)/1
  x(%)->x(m)/1 -> Stimation of spring coefficients/3(dmax1)
  getDeltaXmax1/1(dmax2) -> Stimation of spring coefficients1/5(dmax2_per), x(%)->x(m)1/1
  x(%)->x(m)1/1 -> Stimation of spring coefficients1/4(dmax2)
  x2(m)->x2(%)/1 -> xplot/2, x2/1
  x1(m)->x1(%)/1 -> xplot/1, x1/1
  F2/1 -> Stimation of spring coefficients1/1(F2), Fplot/2, Dynamic muscle 2/3(F2)
  Unit Delay/1 -> Stimation of spring coefficients1/3(Fload)
  Unit Delay1/1 -> Stimation of spring coefficients/2(Fload)
  Unit Delay2/1 -> Rplot/1, Dynamic muscle 2/2(R1)
  Unit Delay3/1 -> Rplot/2, Dynamics muscle 1/3(R2)

== system walkingRobotRL3D/Walking Robot (Angle based)/Antagonistic PAM Left Leg/hipI_pitch PAM/Spring and damping model ==
  F1 : Inport
  F2 : Inport  Port=2
  P1 : Inport  Port=3
  P2 : Inport  Port=4
  Bar->kPa : Gain  Gain=100
  Bar->kPa1 : Gain  Gain=100
  Dynamic muscle 2 : Subsystem
  Dynamics muscle 1 : Subsystem
  Fplot : Scope  NumInputPorts=2
  Pplot : Scope  NumInputPorts=2
  Rplot : Scope  NumInputPorts=2
  Splot : Scope  NumInputPorts=2
  Stimation of spring coefficients : MATLAB Function  TreatAsAtomicUnit=on
  Stimation of spring coefficients1 : MATLAB Function  TreatAsAtomicUnit=on
  Unit Delay{,1..3} (4 alike) : UnitDelay  SampleTime=-1  HasFrameUpgradeWarning=on
  getDeltaXmax : Subsystem
  getDeltaXmax1 : Subsystem
  x(%)->x(m) : Gain  Gain=muscle_nominal_length/100
  x(%)->x(m)1 : Gain  Gain=muscle_nominal_length/100
  x1(m)->x1(%) : Gain  Gain=100/muscle_nominal_length
  x2(m)->x2(%) : Gain  Gain=100/muscle_nominal_length
  xplot : Scope  NumInputPorts=2
  x1 : Outport
  x2 : Outport  Port=2
  wires:
  Dynamics muscle 1/1(R1) -> Unit Delay/1, Unit Delay2/1
  Dynamic muscle 2/1(R2) -> Unit Delay1/1, Unit Delay3/1
  F1/1 -> Stimation of spring coefficients/4(F1), Fplot/1, Dynamics muscle 1/1(F1)
  Dynamic muscle 2/2(x2) -> x2(m)->x2(%)/1
  Dynamics muscle 1/2(x1) -> x1(m)->x1(%)/1
  P1/1 -> Pplot/1, Bar->kPa/1
  Bar->kPa/1 -> Stimation of spring coefficients/1(P1), getDeltaXmax/1(In1)
  P2/1 -> Pplot/2, Bar->kPa1/1
  Bar->kPa1/1 -> getDeltaXmax1/1(In1), Stimation of spring coefficients1/2(P2)
  Stimation of spring coefficients/1(S1) -> Splot/1, Dynamics muscle 1/2(S1)
  Stimation of spring coefficients1/1(S2) -> Splot/2, Dynamic muscle 2/1(S2)
  getDeltaXmax/1(dmax1) -> Stimation of spring coefficients/5(dmax1_per), x(%)->x(m)/1
  x(%)->x(m)/1 -> Stimation of spring coefficients/3(dmax1)
  getDeltaXmax1/1(dmax2) -> Stimation of spring coefficients1/5(dmax2_per), x(%)->x(m)1/1
  x(%)->x(m)1/1 -> Stimation of spring coefficients1/4(dmax2)
  x2(m)->x2(%)/1 -> xplot/2, x2/1
  x1(m)->x1(%)/1 -> xplot/1, x1/1
  F2/1 -> Stimation of spring coefficients1/1(F2), Fplot/2, Dynamic muscle 2/3(F2)
  Unit Delay/1 -> Stimation of spring coefficients1/3(Fload)
  Unit Delay1/1 -> Stimation of spring coefficients/2(Fload)
  Unit Delay2/1 -> Rplot/1, Dynamic muscle 2/2(R1)
  Unit Delay3/1 -> Rplot/2, Dynamics muscle 1/3(R2)

== system walkingRobotRL3D/Walking Robot (Angle based)/Antagonistic PAM Left Leg/hipI_roll PAM/Spring and damping model ==
  F1 : Inport
  F2 : Inport  Port=2
  P1 : Inport  Port=3
  P2 : Inport  Port=4
  Bar->kPa : Gain  Gain=100
  Bar->kPa1 : Gain  Gain=100
  Dynamic muscle 2 : Subsystem
  Dynamics muscle 1 : Subsystem
  Fplot : Scope  NumInputPorts=2
  Pplot : Scope  NumInputPorts=2
  Rplot : Scope  NumInputPorts=2
  Splot : Scope  NumInputPorts=2
  Stimation of spring coefficients : MATLAB Function  TreatAsAtomicUnit=on
  Stimation of spring coefficients1 : MATLAB Function  TreatAsAtomicUnit=on
  Unit Delay{,1..3} (4 alike) : UnitDelay  SampleTime=-1  HasFrameUpgradeWarning=on
  getDeltaXmax : Subsystem
  getDeltaXmax1 : Subsystem
  x(%)->x(m) : Gain  Gain=muscle_nominal_length/100
  x(%)->x(m)1 : Gain  Gain=muscle_nominal_length/100
  x1(m)->x1(%) : Gain  Gain=100/muscle_nominal_length
  x2(m)->x2(%) : Gain  Gain=100/muscle_nominal_length
  xplot : Scope  NumInputPorts=2
  x1 : Outport
  x2 : Outport  Port=2
  wires:
  Dynamics muscle 1/1(R1) -> Unit Delay/1, Unit Delay2/1
  Dynamic muscle 2/1(R2) -> Unit Delay1/1, Unit Delay3/1
  F1/1 -> Stimation of spring coefficients/4(F1), Fplot/1, Dynamics muscle 1/1(F1)
  Dynamic muscle 2/2(x2) -> x2(m)->x2(%)/1
  Dynamics muscle 1/2(x1) -> x1(m)->x1(%)/1
  P1/1 -> Pplot/1, Bar->kPa/1
  Bar->kPa/1 -> Stimation of spring coefficients/1(P1), getDeltaXmax/1(In1)
  P2/1 -> Pplot/2, Bar->kPa1/1
  Bar->kPa1/1 -> getDeltaXmax1/1(In1), Stimation of spring coefficients1/2(P2)
  Stimation of spring coefficients/1(S1) -> Splot/1, Dynamics muscle 1/2(S1)
  Stimation of spring coefficients1/1(S2) -> Splot/2, Dynamic muscle 2/1(S2)
  getDeltaXmax/1(dmax1) -> Stimation of spring coefficients/5(dmax1_per), x(%)->x(m)/1
  x(%)->x(m)/1 -> Stimation of spring coefficients/3(dmax1)
  getDeltaXmax1/1(dmax2) -> Stimation of spring coefficients1/5(dmax2_per), x(%)->x(m)1/1
  x(%)->x(m)1/1 -> Stimation of spring coefficients1/4(dmax2)
  x2(m)->x2(%)/1 -> xplot/2, x2/1
  x1(m)->x1(%)/1 -> xplot/1, x1/1
  F2/1 -> Stimation of spring coefficients1/1(F2), Fplot/2, Dynamic muscle 2/3(F2)
  Unit Delay/1 -> Stimation of spring coefficients1/3(Fload)
  Unit Delay1/1 -> Stimation of spring coefficients/2(Fload)
  Unit Delay2/1 -> Rplot/1, Dynamic muscle 2/2(R1)
  Unit Delay3/1 -> Rplot/2, Dynamics muscle 1/3(R2)

== system walkingRobotRL3D/Walking Robot (Angle based)/Antagonistic PAM Left Leg/kneeI PAM/Spring and damping model ==
  F1 : Inport
  F2 : Inport  Port=2
  P1 : Inport  Port=3
  P2 : Inport  Port=4
  Bar->kPa : Gain  Gain=100
  Bar->kPa1 : Gain  Gain=100
  Dynamic muscle 2 : Subsystem
  Dynamics muscle 1 : Subsystem
  Fplot : Scope  NumInputPorts=2
  Pplot : Scope  NumInputPorts=2
  Rplot : Scope  NumInputPorts=2
  Splot : Scope  NumInputPorts=2
  Stimation of spring coefficients : MATLAB Function  TreatAsAtomicUnit=on
  Stimation of spring coefficients1 : MATLAB Function  TreatAsAtomicUnit=on
  Unit Delay{,1..3} (4 alike) : UnitDelay  SampleTime=-1  HasFrameUpgradeWarning=on
  getDeltaXmax : Subsystem
  getDeltaXmax1 : Subsystem
  x(%)->x(m) : Gain  Gain=muscle_nominal_length/100
  x(%)->x(m)1 : Gain  Gain=muscle_nominal_length/100
  x1(m)->x1(%) : Gain  Gain=100/muscle_nominal_length
  x2(m)->x2(%) : Gain  Gain=100/muscle_nominal_length
  xplot : Scope  NumInputPorts=2
  x1 : Outport
  x2 : Outport  Port=2
  wires:
  Dynamics muscle 1/1(R1) -> Unit Delay/1, Unit Delay2/1
  Dynamic muscle 2/1(R2) -> Unit Delay1/1, Unit Delay3/1
  F1/1 -> Stimation of spring coefficients/4(F1), Fplot/1, Dynamics muscle 1/1(F1)
  Dynamic muscle 2/2(x2) -> x2(m)->x2(%)/1
  Dynamics muscle 1/2(x1) -> x1(m)->x1(%)/1
  P1/1 -> Pplot/1, Bar->kPa/1
  Bar->kPa/1 -> Stimation of spring coefficients/1(P1), getDeltaXmax/1(In1)
  P2/1 -> Pplot/2, Bar->kPa1/1
  Bar->kPa1/1 -> getDeltaXmax1/1(In1), Stimation of spring coefficients1/2(P2)
  Stimation of spring coefficients/1(S1) -> Splot/1, Dynamics muscle 1/2(S1)
  Stimation of spring coefficients1/1(S2) -> Splot/2, Dynamic muscle 2/1(S2)
  getDeltaXmax/1(dmax1) -> Stimation of spring coefficients/5(dmax1_per), x(%)->x(m)/1
  x(%)->x(m)/1 -> Stimation of spring coefficients/3(dmax1)
  getDeltaXmax1/1(dmax2) -> Stimation of spring coefficients1/5(dmax2_per), x(%)->x(m)1/1
  x(%)->x(m)1/1 -> Stimation of spring coefficients1/4(dmax2)
  x2(m)->x2(%)/1 -> xplot/2, x2/1
  x1(m)->x1(%)/1 -> xplot/1, x1/1
  F2/1 -> Stimation of spring coefficients1/1(F2), Fplot/2, Dynamic muscle 2/3(F2)
  Unit Delay/1 -> Stimation of spring coefficients1/3(Fload)
  Unit Delay1/1 -> Stimation of spring coefficients/2(Fload)
  Unit Delay2/1 -> Rplot/1, Dynamic muscle 2/2(R1)
  Unit Delay3/1 -> Rplot/2, Dynamics muscle 1/3(R2)
